simulink model "RobustLateral"  (R2020b)
settings: Solver=VariableStepAuto  StartTime=0.0  StopTime=64  RelTol=1e-3
values from neighbouring files (symbols this model uses):
  A = [-(Cf + Cr)/(m*vx)        -vx + (Cr*Lr - Cf*Lf)/(m*vx) ... (first row only)    [Lab_Lateral.m]
  B = [Cf/m; Lf*Cf/Iz]    [Lab_Lateral.m]
  C = [0 1]    [Lab_Lateral.m]
  Fe = lqr(sysE.a, sysE.b, Qe, Re)    [Lab_Lateral.m]
  Ghinf = inv(sysD.c*inv(eye(2)-sysD.a + sysD.b*Khinf)*sysD.b)    [Lab_Lateral.m]
  Khinf = H_inf_control_design(sysD.a, sysD.b, 0.01*E)    [Lab_Lateral.m]
  L = lqr(A', C', W, V)'    [Lab_Lateral.m]
  m = 1621    [Lab_Lateral.m]
  vx = 10    [Lab_Lateral.m]
undefined symbols (not defined in the file or in its folder): khinf
libraries: simulink x4
settings Model: Creator=DELL  LastModifiedBy=DELL

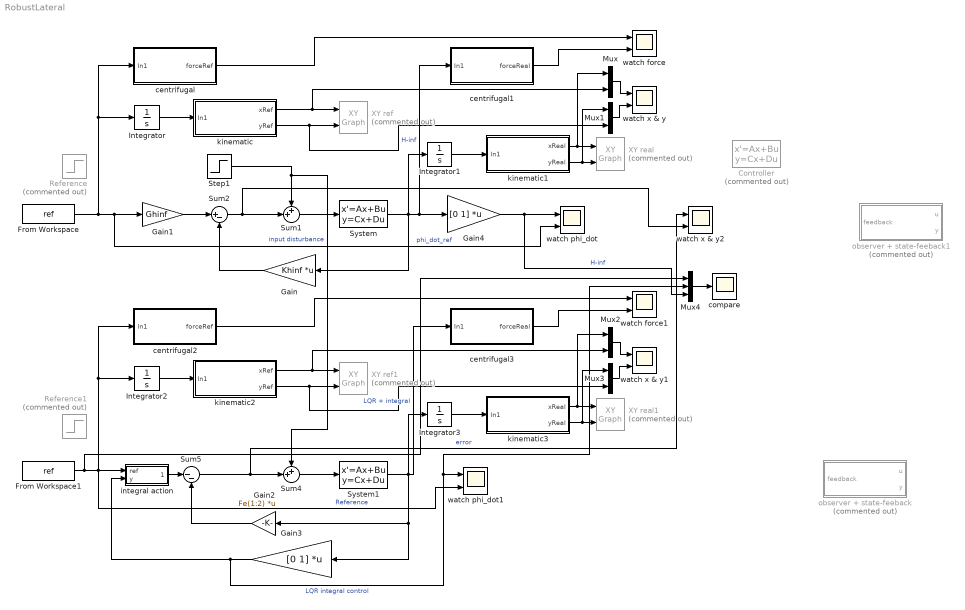
== system RobustLateral ==
  Controller : StateSpace  Commented=on  A=khinf.a  B=khinf.b  C=khinf.c  D=khinf.d  InitialCondition=0
  From Workspace : FromWorkspace  VariableName=ref
  From Workspace1 : FromWorkspace  VariableName=ref
  Gain : Gain  Gain=Khinf  Multiplication=Matrix(K*u) (u vector)
  Gain1 : Gain  Gain=Ghinf
  Gain2 : Gain  Gain=Fe(1:2)  Multiplication=Matrix(K*u) (u vector)
  Gain3 : Gain  Gain=[0 1]  Multiplication=Matrix(K*u) (u vector)
  Gain4 : Gain  Gain=[0 1]  Multiplication=Matrix(K*u) (u vector)
  Integrator{,1..3} (4 alike) : Integrator
  Mux{,1..3} (4 alike) : Mux  Inputs=2
  Mux4 : Mux  Inputs=3
  Reference : Step  Commented=on  SampleTime=0
  Reference1 : Step  Commented=on  SampleTime=0
  Step1 : Step  Time=2  After=0.02  SampleTime=0
  Sum1 : Sum  Inputs=++|
  Sum2 : Sum  Inputs=|+-
  Sum4 : Sum  Inputs=++|
  Sum5 : Sum  Inputs=|--
  System : StateSpace  A=A  B=B  C=eye(2)  D=[0; 0]  InitialCondition=0
  System1 : StateSpace  A=A  B=B  C=eye(2)  D=[0; 0]  InitialCondition=0
  XY real : simulink/Sinks/XY Graph  Commented=on  xmin=0  xmax=400  ymin=0  ymax=350  st=ts
  XY real1 : simulink/Sinks/XY Graph  Commented=on  xmin=0  xmax=400  ymin=0  ymax=350  st=ts
  XY ref : simulink/Sinks/XY Graph  Commented=on  xmin=0  xmax=400  ymin=0  ymax=350  st=ts
  XY ref1 : simulink/Sinks/XY Graph  Commented=on  xmin=0  xmax=400  ymin=0  ymax=350  st=ts
  centrifugal : Subsystem
  centrifugal1 : Subsystem
  centrifugal2 : Subsystem
  centrifugal3 : Subsystem
  compare : Scope
  integral action : Subsystem
  kinematic : Subsystem
  kinematic1 : Subsystem
  kinematic2 : Subsystem
  kinematic3 : Subsystem
  observer + state-feeback : Subsystem  Commented=on
  observer + state-feeback1 : Subsystem  Commented=on
  watch force : Scope  NumInputPorts=2
  watch force1 : Scope  NumInputPorts=2
  watch phi_dot : Scope  NumInputPorts=2
  watch phi_dot1 : Scope  NumInputPorts=2
  watch x & y : Scope  NumInputPorts=2
  watch x & y1 : Scope  NumInputPorts=2
  watch x & y2 : Scope  NumInputPorts=2
  wires:
  From Workspace/1 -> centrifugal/1(In1), Integrator/1, Gain1/1, watch phi_dot/2  "phi_dot_ref"
  Sum2/1 -> watch x & y2/2, Sum1/2
  Sum1/1 -> System/1
  Step1/1 -> Sum4/1, Sum1/1  "input disturbance"
  System/1 -> Gain4/1, centrifugal1/1(In1), Integrator1/1, Gain/1  "H-inf"
  Integrator/1 -> kinematic/1(In1)
  Integrator1/1 -> kinematic1/1(In1)
  kinematic/1(xRef) -> Mux/2, XY ref/1
  kinematic/2(yRef) -> Mux1/2, XY ref/2
  kinematic1/1(xReal) -> Mux/1, XY real/1
  kinematic1/2(yReal) -> Mux1/1, XY real/2
  Mux/1 -> watch x & y/1
  Mux1/1 -> watch x & y/2
  centrifugal/1(forceRef) -> watch force/1
  centrifugal1/1(forceReal) -> watch force/2
  centrifugal3/1(forceReal) -> watch force1/2
  centrifugal2/1(forceRef) -> watch force1/1
  Mux3/1 -> watch x & y1/2
  kinematic3/2(yReal) -> Mux3/1, XY real1/2
  kinematic3/1(xReal) -> Mux2/1, XY real1/1
  kinematic2/1(xRef) -> Mux2/2, XY ref1/1
  Mux2/1 -> watch x & y1/1
  kinematic2/2(yRef) -> Mux3/2, XY ref1/2
  Sum4/1 -> System1/1
  Integrator2/1 -> kinematic2/1(In1)
  Sum5/1 -> watch x & y2/1, Sum4/2  "error"
  System1/1 -> Gain3/1, Gain2/1, centrifugal3/1(In1), Integrator3/1  "LQR + integral"
  From Workspace1/1 -> Mux4/1, watch phi_dot1/2, integral action/1(ref), centrifugal2/1(In1), Integrator2/1  "Reference"
  Integrator3/1 -> kinematic3/1(In1)
  integral action/1(integral) -> Sum5/1
  Gain/1 -> Sum2/2
  Gain2/1 -> Sum5/2
  Gain3/1 -> Mux4/2, watch phi_dot1/1, integral action/2(y)  "LQR integral control"
  Gain4/1 -> Mux4/3, watch phi_dot/1  "H-inf"
  Gain1/1 -> Sum2/1
  Mux4/1 -> compare/1

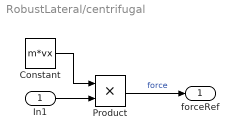
== system RobustLateral/centrifugal ==
  In1 : Inport
  Constant : Constant  Value=m*vx
  Product : Product
  forceRef : Outport
  wires:
  In1/1 -> Product/2
  Constant/1 -> Product/1
  Product/1 -> forceRef/1  "force"

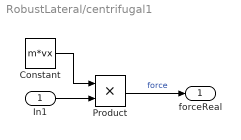
== system RobustLateral/centrifugal1 ==
  In1 : Inport
  Constant : Constant  Value=m*vx
  Product : Product
  forceReal : Outport
  wires:
  In1/1 -> Product/2
  Constant/1 -> Product/1
  Product/1 -> forceReal/1  "force"

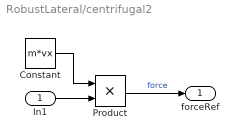
== system RobustLateral/centrifugal2 ==
  In1 : Inport
  Constant : Constant  Value=m*vx
  Product : Product
  forceRef : Outport
  wires:
  In1/1 -> Product/2
  Constant/1 -> Product/1
  Product/1 -> forceRef/1  "force"

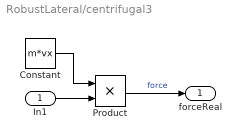
== system RobustLateral/centrifugal3 ==
  In1 : Inport
  Constant : Constant  Value=m*vx
  Product : Product
  forceReal : Outport
  wires:
  In1/1 -> Product/2
  Constant/1 -> Product/1
  Product/1 -> forceReal/1  "force"

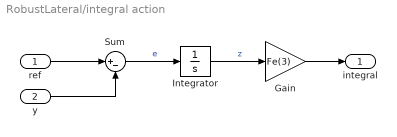
== system RobustLateral/integral action ==
  ref : Inport
  y : Inport  Port=2
  Gain : Gain  Gain=Fe(3)
  Integrator : Integrator
  Sum : Sum  Inputs=|+-
  integral : Outport
  wires:
  ref/1 -> Sum/1
  y/1 -> Sum/2
  Sum/1 -> Integrator/1  "e"
  Integrator/1 -> Gain/1  "z"
  Gain/1 -> integral/1

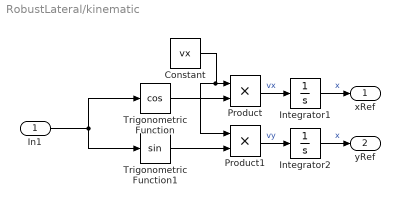
== system RobustLateral/kinematic ==
  In1 : Inport
  Constant : Constant  Value=vx
  Integrator1 : Integrator
  Integrator2 : Integrator
  Product : Product
  Product1 : Product
  Trigonometric Function : Trigonometry  Operator=cos
  Trigonometric Function1 : Trigonometry
  xRef : Outport
  yRef : Outport  Port=2
  wires:
  In1/1 -> Trigonometric Function1/1, Trigonometric Function/1
  Trigonometric Function1/1 -> Product1/2
  Trigonometric Function/1 -> Product/2
  Constant/1 -> Product1/1, Product/1
  Product/1 -> Integrator1/1  "vx"
  Integrator1/1 -> xRef/1  "x"
  Product1/1 -> Integrator2/1  "vy"
  Integrator2/1 -> yRef/1  "x"

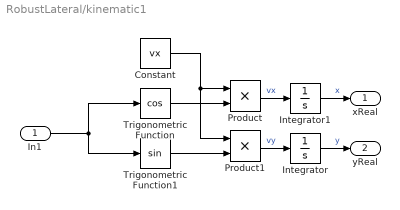
== system RobustLateral/kinematic1 ==
  In1 : Inport
  Constant : Constant  Value=vx
  Integrator : Integrator
  Integrator1 : Integrator
  Product : Product
  Product1 : Product
  Trigonometric Function : Trigonometry  Operator=cos
  Trigonometric Function1 : Trigonometry
  xReal : Outport
  yReal : Outport  Port=2
  wires:
  In1/1 -> Trigonometric Function1/1, Trigonometric Function/1
  Trigonometric Function1/1 -> Product1/2
  Trigonometric Function/1 -> Product/2
  Constant/1 -> Product1/1, Product/1
  Product/1 -> Integrator1/1  "vx"
  Integrator1/1 -> xReal/1  "x"
  Product1/1 -> Integrator/1  "vy"
  Integrator/1 -> yReal/1  "y"

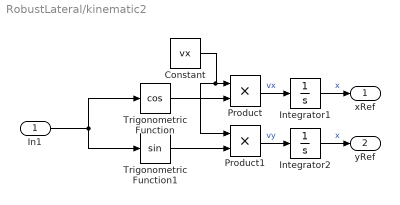
== system RobustLateral/kinematic2 ==
  In1 : Inport
  Constant : Constant  Value=vx
  Integrator1 : Integrator
  Integrator2 : Integrator
  Product : Product
  Product1 : Product
  Trigonometric Function : Trigonometry  Operator=cos
  Trigonometric Function1 : Trigonometry
  xRef : Outport
  yRef : Outport  Port=2
  wires:
  In1/1 -> Trigonometric Function1/1, Trigonometric Function/1
  Trigonometric Function1/1 -> Product1/2
  Trigonometric Function/1 -> Product/2
  Constant/1 -> Product1/1, Product/1
  Product/1 -> Integrator1/1  "vx"
  Integrator1/1 -> xRef/1  "x"
  Product1/1 -> Integrator2/1  "vy"
  Integrator2/1 -> yRef/1  "x"

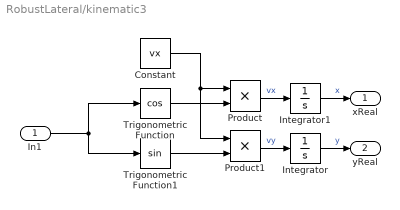
== system RobustLateral/kinematic3 ==
  In1 : Inport
  Constant : Constant  Value=vx
  Integrator : Integrator
  Integrator1 : Integrator
  Product : Product
  Product1 : Product
  Trigonometric Function : Trigonometry  Operator=cos
  Trigonometric Function1 : Trigonometry
  xReal : Outport
  yReal : Outport  Port=2
  wires:
  In1/1 -> Trigonometric Function1/1, Trigonometric Function/1
  Trigonometric Function1/1 -> Product1/2
  Trigonometric Function/1 -> Product/2
  Constant/1 -> Product1/1, Product/1
  Product/1 -> Integrator1/1  "vx"
  Integrator1/1 -> xReal/1  "x"
  Product1/1 -> Integrator/1  "vy"
  Integrator/1 -> yReal/1  "y"

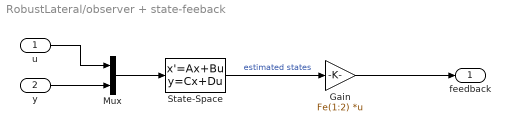
== system RobustLateral/observer + state-feeback ==
  u : Inport
  y : Inport  Port=2
  Gain : Gain  Gain=Fe(1:2)  Multiplication=Matrix(K*u) (u vector)
  Mux : Mux  Inputs=2
  State-Space : StateSpace  A=A - L*C  B=[B L]  C=eye(2)  D=zeros(2, 2)  InitialCondition=0
  feedback : Outport
  wires:
  u/1 -> Mux/1
  y/1 -> Mux/2
  Mux/1 -> State-Space/1
  State-Space/1 -> Gain/1  "estimated states"
  Gain/1 -> feedback/1

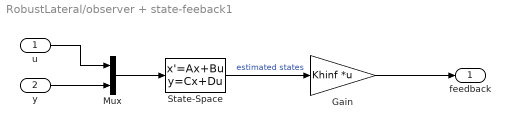
== system RobustLateral/observer + state-feeback1 ==
  u : Inport
  y : Inport  Port=2
  Gain : Gain  Gain=Khinf  Multiplication=Matrix(K*u) (u vector)
  Mux : Mux  Inputs=2
  State-Space : StateSpace  A=A - L*C  B=[B L]  C=eye(2)  D=zeros(2, 2)  InitialCondition=0
  feedback : Outport
  wires:
  u/1 -> Mux/1
  y/1 -> Mux/2
  Mux/1 -> State-Space/1
  State-Space/1 -> Gain/1  "estimated states"
  Gain/1 -> feedback/1
